simulink model "sampleModel359"  (R2021b)
settings: Solver=VariableStepAuto  StartTime=0.0  StopTime=10.0  RelTol=1e-3
undefined symbols (not defined in the file or in its folder): DiscIntNeverNeededParam
libraries: simulink x2
settings Model: Creator=user  LastModifiedBy=user

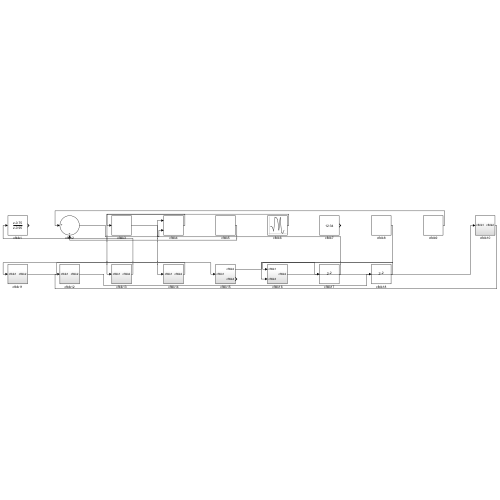
[thumbnail: Simulink's stored preview of the top-level diagram]
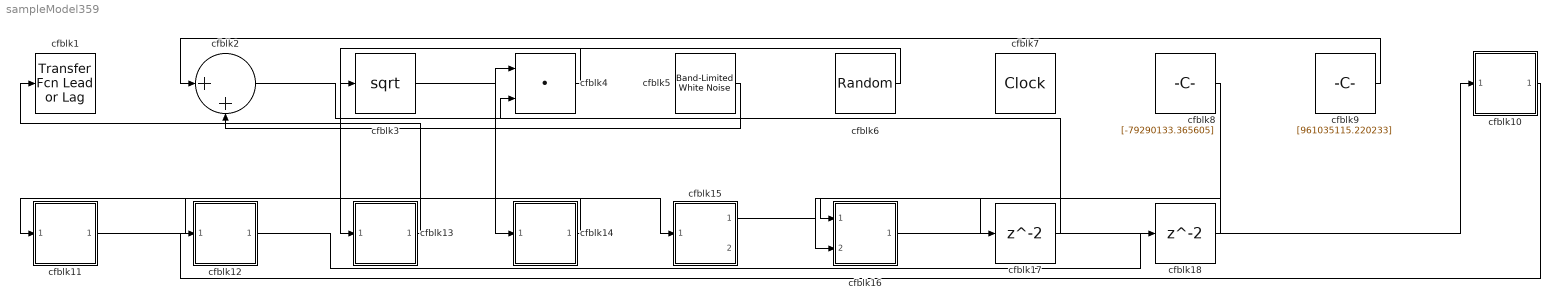
== system sampleModel359 ==
  cfblk1 : simulink/Discrete/Transfer Fcn Lead or Lag  PoleZ=0.95  ZeroZ=0.75  ICPrevOutput=0.0  ICPrevInput=0.0  DoSatur=off
      settings: SourceProductBaseCode=SL
  cfblk10 : Subsystem
  cfblk11 : Subsystem
  cfblk12 : Subsystem
  cfblk13 : Subsystem
  cfblk14 : Subsystem
  cfblk15 : Subsystem
  cfblk16 : Subsystem
  cfblk17 : Delay  SampleTime=1
  cfblk18 : Delay  SampleTime=1
  cfblk2 : Sum  Inputs=|++
  cfblk3 : Sqrt  SaturateOnIntegerOverflow=on
  cfblk4 : DotProduct  InputSameDT=on  OutDataTypeStr=Inherit: Inherit via internal rule
  cfblk5 : simulink/Sources/Band-Limited White Noise  Cov=[4079980656.623296]  Ts=0.1  seed=[2401078555.000000]
  cfblk6 : RandomNumber  Mean=[-70148.763672]  Variance=[28240.553787]  Seed=[4735454.000000]  SampleTime=0.1
  cfblk7 : DigitalClock
  cfblk8 : Constant  Value=[-79290133.365605]  SampleTime=1
  cfblk9 : Constant  Value=[961035115.220233]  SampleTime=1
  wires:
  cfblk6/1 -> cfblk13/1(cfblk1)
  cfblk4/1 -> cfblk3/1
  cfblk11/1(cfblk2) -> cfblk15/1(cfblk1)
  cfblk2/1 -> cfblk4/2
  cfblk8/1 -> cfblk16/2(cfblk3)
  cfblk9/1 -> cfblk2/1
  cfblk10/1(cfblk2) -> cfblk12/1(cfblk1)
  cfblk16/1(cfblk2) -> cfblk10/1(cfblk1)
  cfblk14/1(cfblk2) -> cfblk11/1(cfblk1)
  cfblk13/1(cfblk2) -> cfblk1/1
  cfblk3/1 -> cfblk14/1(cfblk1)
  cfblk5/1 -> cfblk2/2
  cfblk15/1(cfblk2) -> cfblk17/1
  cfblk17/1 -> cfblk4/1
  cfblk12/1(cfblk2) -> cfblk18/1
  cfblk18/1 -> cfblk16/1(cfblk1)

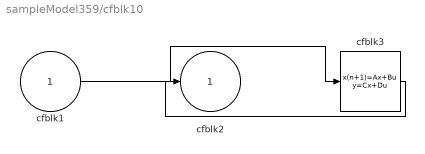
== system sampleModel359/cfblk10 ==
  cfblk1 : Inport
  cfblk3 : DiscreteStateSpace
  cfblk2 : Outport
  wires:
  cfblk1/1 -> cfblk3/1
  cfblk3/1 -> cfblk2/1

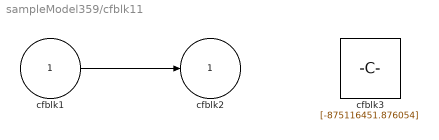
== system sampleModel359/cfblk11 ==
  cfblk1 : Inport
  cfblk3 : Constant  Value=[-875116451.876054]  SampleTime=1
  cfblk2 : Outport
  wires:
  cfblk1/1 -> cfblk2/1

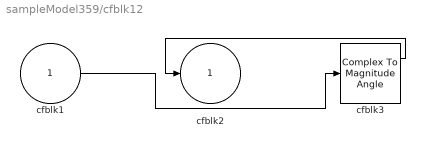
== system sampleModel359/cfblk12 ==
  cfblk1 : Inport
  cfblk3 : ComplexToMagnitudeAngle
  cfblk2 : Outport
  wires:
  cfblk3/1 -> cfblk2/1
  cfblk1/1 -> cfblk3/1

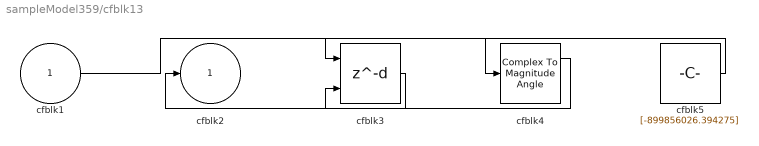
== system sampleModel359/cfblk13 ==
  cfblk1 : Inport
  cfblk3 : Delay  DelayLengthSource=Input port  SampleTime=1
      settings: InputPortMap=u0,p1
  cfblk4 : ComplexToMagnitudeAngle
  cfblk5 : Constant  Value=[-899856026.394275]  SampleTime=1
  cfblk2 : Outport
  wires:
  cfblk5/1 -> cfblk3/1
  cfblk3/1 -> cfblk2/1
  cfblk4/1 -> cfblk3/2
  cfblk1/1 -> cfblk4/1

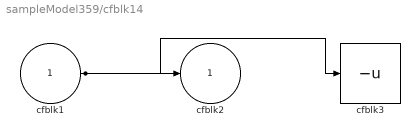
== system sampleModel359/cfblk14 ==
  cfblk1 : Inport
  cfblk3 : UnaryMinus
  cfblk2 : Outport
  wires:
  cfblk1/1 -> cfblk2/1, cfblk3/1

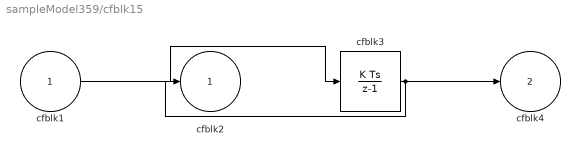
== system sampleModel359/cfblk15 ==
  cfblk1 : Inport
  cfblk3 : DiscreteIntegrator  ICPrevOutput=DiscIntNeverNeededParam  ICPrevScaledInput=DiscIntNeverNeededParam
  cfblk2 : Outport
  cfblk4 : Outport  Port=2
  wires:
  cfblk1/1 -> cfblk3/1
  cfblk3/1 -> cfblk2/1, cfblk4/1

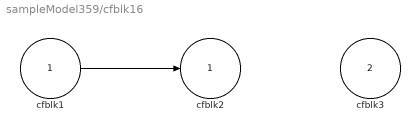
== system sampleModel359/cfblk16 ==
  cfblk1 : Inport
  cfblk3 : Inport  Port=2
  cfblk2 : Outport
  wires:
  cfblk1/1 -> cfblk2/1
